simulink model "Test_Nonlinear_system"  (R2022b)
settings: Solver=VariableStepAuto  StartTime=0.0  StopTime=50  RelTol=1e-3
values from neighbouring files (symbols this model uses):
  A = double(A)    [sys_Modelling.m]
  B = double(B)    [sys_Modelling.m]
  C = zeros((N+1)*n, N*p)    [MPC_Matrices.m]    (also in sys_Modelling.m = double(C))
  L = place(sys.A', sys.C',ew_L)'    [Controller_Observer.m]    (also in LQR_Luenberger.m)
undefined symbols (not defined in the file or in its folder): K_neu, u_ap, V_neu
libraries: simulink_extras x2
settings Model: Creator=renzhijian  LastModifiedBy=12056

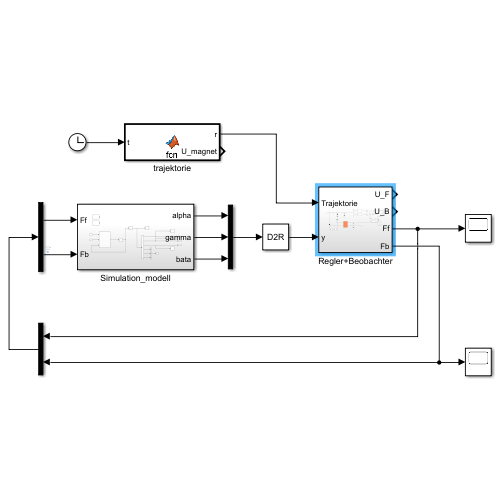
[thumbnail: Simulink's stored preview of the top-level diagram]
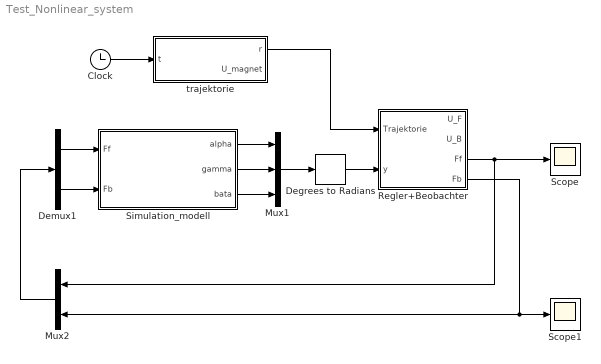
== system Test_Nonlinear_system ==
  Clock : Clock
  Degrees to Radians : simulink_extras/Transformations/Degrees to Radians
  Demux1 : Demux  Outputs=2
  Mux1 : Mux  Inputs=3
  Mux2 : Mux  Inputs=2
  Regler+Beobachter : Subsystem
  Scope : Scope
  Scope1 : Scope
  Simulation_modell : Subsystem
  trajektorie : MATLAB Function  TreatAsAtomicUnit=on
  wires:
  Mux2/1 -> Demux1/1
  Simulation_modell/2(gamma) -> Mux1/2
  Simulation_modell/1(alpha) -> Mux1/1
  Simulation_modell/3(bata) -> Mux1/3
  Regler+Beobachter/3(Ff) -> Scope/1, Mux2/1
  Regler+Beobachter/4(Fb) -> Scope1/1, Mux2/2
  Demux1/1 -> Simulation_modell/1(Ff)
  Demux1/2 -> Simulation_modell/2(Fb)
  Clock/1 -> trajektorie/1(t)
  Mux1/1 -> Degrees to Radians/1
  Degrees to Radians/1 -> Regler+Beobachter/2(y)
  trajektorie/1(r) -> Regler+Beobachter/1(Trajektorie)

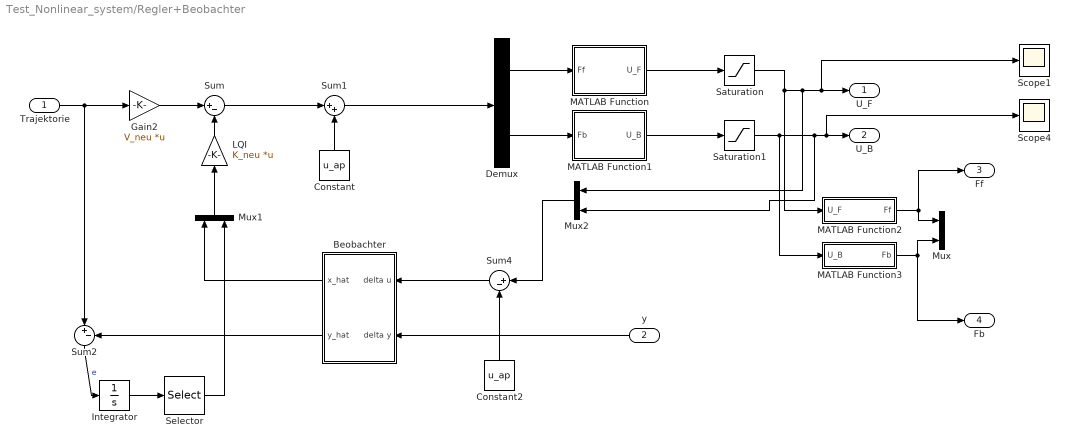
== system Test_Nonlinear_system/Regler+Beobachter ==
  Trajektorie : Inport
  y : Inport  Port=2
  Beobachter : Subsystem
  Constant : Constant  Value=u_ap
  Constant2 : Constant  Value=u_ap
  Demux : Demux  Outputs=2
  Gain2 : Gain  Gain=V_neu  Multiplication=Matrix(K*u) (u vector)
  Integrator : Integrator
  LQI : Gain  Gain=K_neu  Multiplication=Matrix(K*u) (u vector)
  MATLAB Function : MATLAB Function  TreatAsAtomicUnit=on
  MATLAB Function1 : MATLAB Function  TreatAsAtomicUnit=on
  MATLAB Function2 : MATLAB Function  TreatAsAtomicUnit=on
  MATLAB Function3 : MATLAB Function  TreatAsAtomicUnit=on
  Mux : Mux  Inputs=2
  Mux1 : Mux  Inputs=2
  Mux2 : Mux  Inputs=2
  Saturation : Saturate  UpperLimit=4  LowerLimit=0
  Saturation1 : Saturate  UpperLimit=4  LowerLimit=0
  Scope1 : Scope
  Scope4 : Scope
  Selector : Selector  InputPortWidth=3  IndexOptions=Index vector (dialog)  Indices=[1 2]  OutputSizes=1
  Sum : Sum  Inputs=|+-
  Sum1 : Sum  Inputs=|++
  Sum2 : Sum  Inputs=|+-
  Sum4 : Sum  Inputs=|+-
  U_F : Outport
  U_B : Outport  Port=2
  Ff : Outport  Port=3
  Fb : Outport  Port=4
  wires:
  MATLAB Function1/1(U_B) -> Saturation1/1
  y/1 -> Beobachter/2(delta y)
  Saturation1/1 -> Mux2/2, Scope4/1, U_B/1, MATLAB Function3/1(U_B)
  Demux/1 -> MATLAB Function/1(Ff)
  Sum1/1 -> Demux/1
  Saturation/1 -> Mux2/1, Scope1/1, U_F/1, MATLAB Function2/1(U_F)
  MATLAB Function2/1(Ff) -> Ff/1, Mux/1
  MATLAB Function3/1(Fb) -> Fb/1, Mux/2
  Constant2/1 -> Sum4/2
  Constant/1 -> Sum1/2
  MATLAB Function/1(U_F) -> Saturation/1
  Sum4/1 -> Beobachter/1(delta u)
  Demux/2 -> MATLAB Function1/1(Fb)
  Trajektorie/1 -> Gain2/1, Sum2/1
  Sum/1 -> Sum1/1
  Sum2/1 -> Integrator/1  "e"
  Integrator/1 -> Selector/1
  Beobachter/2(y_hat) -> Sum2/2
  Beobachter/1(x_hat) -> Mux1/1
  Mux1/1 -> LQI/1
  LQI/1 -> Sum/2
  Gain2/1 -> Sum/1
  Selector/1 -> Mux1/2
  Mux2/1 -> Sum4/1

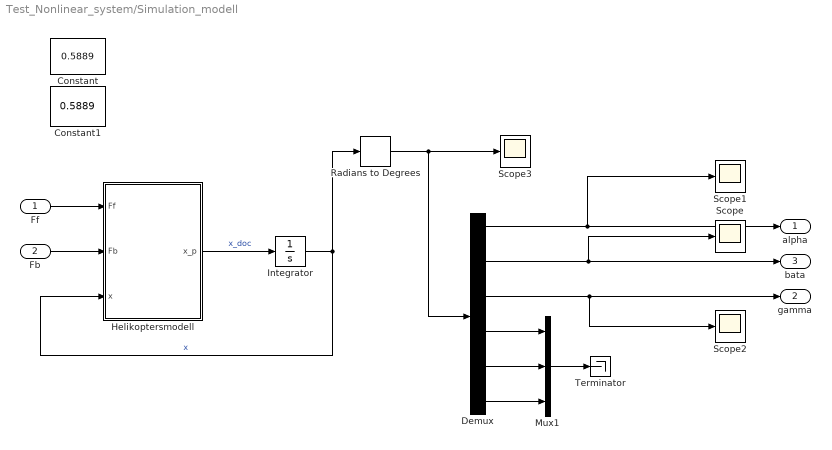
== system Test_Nonlinear_system/Simulation_modell ==
  Ff : Inport
  Fb : Inport  Port=2
  Constant : Constant  Value=0.5889
  Constant1 : Constant  Value=0.5889
  Demux : Demux  Outputs=6
  Helikoptersmodell : MATLAB Function  TreatAsAtomicUnit=on
  Integrator : Integrator  InitialCondition=[0;-27*pi/180;0;0;0;0]
  Mux1 : Mux  Inputs=3
  Radians to Degrees : simulink_extras/Transformations/Radians to Degrees
  Scope{,1..3} (4 alike) : Scope
  Terminator : Terminator
  alpha : Outport  VectorParamsAs1DForOutWhenUnconnected=off
  gamma : Outport  Port=2  VectorParamsAs1DForOutWhenUnconnected=off
  bata : Outport  Port=3  VectorParamsAs1DForOutWhenUnconnected=off
  wires:
  Mux1/1 -> Terminator/1
  Integrator/1 -> Radians to Degrees/1, Helikoptersmodell/3(x)  "x"
  Demux/3 -> Scope2/1, gamma/1
  Radians to Degrees/1 -> Scope3/1, Demux/1
  Demux/4 -> Mux1/1
  Helikoptersmodell/1(x_p) -> Integrator/1  "x_doc"
  Demux/5 -> Mux1/2
  Demux/1 -> Scope1/1, alpha/1
  Demux/2 -> bata/1, Scope/1
  Demux/6 -> Mux1/3
  Ff/1 -> Helikoptersmodell/1(Ff)
  Fb/1 -> Helikoptersmodell/2(Fb)

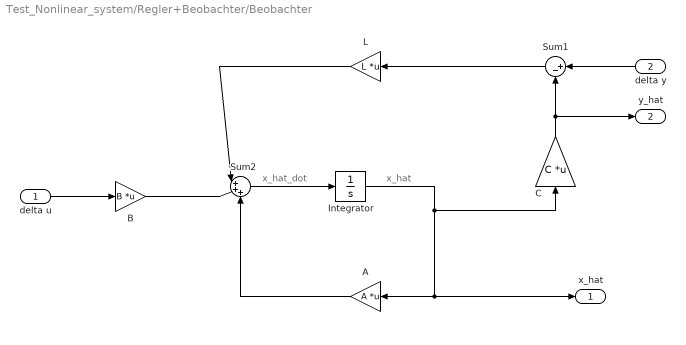
== system Test_Nonlinear_system/Regler+Beobachter/Beobachter ==
  note: x_hat_dot
  note: x_hat
  delta u : Inport
  delta y : Inport  Port=2
  A : Gain  Gain=A  Multiplication=Matrix(K*u) (u vector)
  B : Gain  Gain=B  Multiplication=Matrix(K*u) (u vector)
  C : Gain  Gain=C  Multiplication=Matrix(K*u) (u vector)
  Integrator : Integrator  InitialCondition=[0;-27*pi/180;0;0;0;0]
  L : Gain  Gain=L  Multiplication=Matrix(K*u) (u vector)
  Sum1 : Sum  Inputs=|+-
  Sum2 : Sum  Inputs=|+++
  x_hat : Outport
  y_hat : Outport  Port=2
  wires:
  Integrator/1 -> A/1, x_hat/1, C/1
  L/1 -> Sum2/1
  Sum2/1 -> Integrator/1
  delta u/1 -> B/1
  Sum1/1 -> L/1
  A/1 -> Sum2/3
  B/1 -> Sum2/2
  delta y/1 -> Sum1/1
  C/1 -> Sum1/2, y_hat/1

== matlab function Test_Nonlinear_system/Simulation_modell/Helikoptersmodell ==
  data: Ff input; x_p output; Fb input; x input
function x_p = fcn(Ff, Fb, x)
alpha = x(1);
beta = x(2);
gamma = x(3);
alphadot = x(4);
betadot = x(5);
gammadot = x(6);
%Helikopterseigenschaft
l1 = 0.655; %Distance between travel axis to helicopter body  
l2 = 0.262; %Length of the secondary arm
l3 = 0.1355; %Force arm of the gravity of secondary arm
l4 = 0.2285; %Length from Joint 1 to crossing point
l5 = 0.21; %Length from Joint 1 to midpoint of main arm 
l6 = 0.355/2; %Distance between pitch to each motor 
l7 = 0.534;
h = 0.042+0.019/2; % Distance between axis Y and main arm

%Gewicht
mw = 1.918;%Mass of the counterweight
marm2 = 0.138;%Mass of secondary arm
marm1 = 0.377;%Mass of main arm
mf = 0.661;%Mass of front motor and bodies
mb = 0.661;%Mass of back motor and bodies
mj2 = 0.106;%Mass of the joint2
mmag = 0.07;%Mass of the magnet
g = 9.81;%Erdbeschleunigung
theta = deg2rad(15);%Crossing angle of main and secondary arm
phi = 0.1427;%Deviation of the helicopter relative to joint2
d = 0.102;%Distance between joint3 to the rail

%% MOMENT OF INERTIA
%% beta
J_mw = (1/12)*mw*(0.070^2 + 0.057^2);
J_marm1 = (1/12)*marm1*(0.915^2 + 0.019^2);
J_marm2 = (1/12)*marm2*(0.305^2 + 0.025^2);

Jbeta = J_mw + mw * ((l4+l2*cos(theta))^2+(l2*sin(theta)-h)^2) ...,       % Moment of CounterWeight
    + J_marm1 + marm1 * (((l5)/2)^2+h^2) ...,                               % Moment of main arm
    + J_marm2 + marm2 * (((l3*cos(theta))+l4)^2+(l3*sin(theta)-h)^2) ...,   % Moment of secondary arm
    + (mf+mb)*(l1^2+(0.044+h)^2) ...,                                       % Moment of heli(simplify)
    + mj2*(l1^2+(h+0.019+0.028)^2) ...,                                     % Moment of joint 2
    + mmag*(l7^2+(h+0.062*sin(pi/3))^2);                                    % Moment of Magnet
% 1.1435        1.1708

%% gamma
J_body  =   1/12*0.2*(3*0.114^2 + 0.027^2);           % Body = Cylinder
J_moter =   1/12*0.287*(3*0.0195^2 + 0.069^2);        % Motor = Cylinder
J_bar   =   1/12*0.322*(0.495^2 + 0.006^2);           % Bar = Cubic
J_joint =   1/12*0.026*(0.019^2 + 0.025^2);           % joint = Cubic

Jgamma = 2*(J_body+0.2*((0.027/2+0.069-0.041)^2+(0.355/2)^2))+ ...,           % Moment of bodies
    2*(J_moter+0.287*((0.041-0.069/2)^2+(0.355/2)^2))+ ...,                     % Moment of Motors
    J_bar+0.322*(0.041+0.006/2)^2+ ...,                                         % Moment of bar
    J_joint+0.026*(0.041-0.019/2)^2;                                            % Moment of joints3
% 0.0402        0.0554

%% alpha    simplify
% modification
aRb = [cos(beta) 0 sin(beta); 
    0 1 0; 
    -sin(beta) 0 cos(beta)];
bRc = [cos(gamma) -sin(gamma) 0; 
    sin(gamma) cos(gamma) 0; 
    0 0 1];
arb = [l1*sin(beta); 0; l1*cos(beta)];

cP_f = [-0.065; -l6; 0];
cP_b = [-0.065; l6; 0];

aP_f = aRb*bRc*cP_f + arb;
aP_b = aRb*bRc*cP_b + arb;

D_Pf = aP_f(2)^2 + aP_f(3)^2;
D_Pb = aP_b(2)^2 + aP_b(3)^2;


J_mw_alpha = (1/12)*mw*((0.070^2 + 0.057^2)*(sin((pi/2)+beta-theta))^2+(0.057^2 + 0.057^2)*(cos((pi/2)+beta-theta))^2);
J_marm1_alpha = (1/12)*marm1*((0.915^2+0.019^2)*(cos(beta))^2+(0.019^2+0.019^2)*(sin(beta))^2);
J_marm2_alpha = (1/12)*marm2*((0.305^2+0.025^2)*(cos(beta-theta))^2 +(0.025^2+0.025^2)*(sin(beta-theta))^2);
J_j1_alpha = 1/12*0.029*((0.019^2 + 0.025^2)*(cos(beta))^2 + (0.019^2 + 0.019^2)*(sin(beta))^2);
J_bar_alpha =  1/12*0.322*((0.495^2 + 0.006^2)*((cos(beta))^2+(cos(gamma))^2) + (0.006^2 + 0.006^2)*(sin(beta))^2);
J_joint_alpha =   1/12*0.026*((0.019^2 + 0.025^2)*((cos(beta))^2+(cos(gamma))^2) + (0.019^2 + 0.019^2)*(sin(beta))^2);
J_body_alpha = 1/12*0.2*(3*0.114^2 + 0.027^2)*((sin(beta))^2+(cos(gamma))^2) + 1/2*0.2*0.114^2*(cos(beta))^2; 
J_moter_alpha =   1/12*0.287*(3*0.0195^2 + 0.069^2)*((sin(beta))^2+(cos(gamma))^2) + 1/2*0.287*0.0195^2*(cos(beta))^2;

Jalpha = J_mw_alpha + mw*((l4*cos(beta)+l2*cos(theta-beta))^2) ...,                  % Moment of CounterWeight
    + J_marm1_alpha + marm1*(l5*cos(beta))^2 ...,                                    % Moment of main arm
    + J_marm2_alpha + marm2*((l3*cos(theta-beta)+l4*cos(beta))^2)...,               % Moment of secondary arm
    + mj2*(l1*cos(beta))^2 ...,                                                % Moment of joint2
    + mmag*(l7*cos(beta))^2 ...,                                               % Moment of magnet
    + J_j1_alpha + 0.029*((0.042-0.019/2)*sin(beta))^2 ...,                          % Moment of joint1
    + J_bar_alpha + 0.322*(l1*cos(beta)+(0.042+0.019+0.028+0.041+0.006/2)*sin(beta))^2 ...,  % Moment of bar
    + J_joint_alpha + 0.026*(l1*cos(beta)+(0.042+0.019+0.028+0.041-0.019/2)*sin(beta))^2 ...,% Moment of joint3
    + 2*J_body_alpha + 2*J_moter_alpha + (0.2+0.287)*(D_Pf+D_Pb);                           % Moment of Motors and Bodies
% 1.1794

%% MOMENT
%% alpha
Malpha = -(Ff+Fb)*sin(gamma)*l1*cos(beta);

%% beta
M_all = (mw*g*(l2*cos(theta)+l4) + marm2*g*(l3*cos(theta)+l4) - (mf+mb+mj2)*g*l1 - marm1*g*l5 -mmag*g*l7)*cos(0);
mass_position = M_all / ((mw+marm2+marm1+mmag+mj2+mf+mb)*g);
Mbeta = (Ff+Fb)*l1*cos(gamma) + (mw+marm2+marm1+mmag+mj2+mf+mb)*g*(mass_position*cos(beta)-h*sin(beta));

%% gamma
Mgamma = (Ff-Fb)*l6 + mb*g*cos(phi+gamma)*l6/cos(phi) - mf*g*cos(phi-gamma)*l6/cos(phi);




%% SOLVE
alphadot_2 = Malpha/Jalpha;
betadot_2 = Mbeta/Jbeta;        % 1.1435
gammadot_2 = Mgamma/Jgamma;     % 0.0402


x_p = [alphadot;
    betadot;
    gammadot;
    alphadot_2;
    betadot_2;
    gammadot_2
    ];
x_p(1:3) = x(4:6);
x_p(4) = alphadot_2;
x_p(5) = betadot_2;
x_p(6) = gammadot_2;

== matlab function Test_Nonlinear_system/Regler+Beobachter/MATLAB Function ==
  data: Ff input; U_F output
function U_F = fcn(Ff)
 U_F= (10000/733*abs(Ff))^(1/2);
end

== matlab function Test_Nonlinear_system/Regler+Beobachter/MATLAB Function1 ==
  data: Fb input; U_B output
function U_B = fcn(Fb)
 U_B= sqrt(1000/66*abs(Fb));
end

== matlab function Test_Nonlinear_system/Regler+Beobachter/MATLAB Function2 ==
  data: U_F input; Ff output
function Ff = fcn(U_F)
Ff = 0.0733*U_F^2;
end

== matlab function Test_Nonlinear_system/Regler+Beobachter/MATLAB Function3 ==
  data: U_B input; Fb output
function Fb = fcn(U_B)
 Fb = 0.066*U_B^2;
end

== matlab function Test_Nonlinear_system/trajektorie ==
  data: t input; r output; U_magnet output
function [r, U_magnet] = fcn(t)
beta = -27;
if t <= 10
    a0 = five_times_plan(0, -27, 0, 0, 10, 0, 0, 0);
    alpha = 0;
    beta = a0(1)+a0(2)*t+a0(3)*t^2+a0(4)*t^3+a0(5)*t^4+a0(6)*t^5;
    U_magnet = 0;
elseif t > 10 && t <= 18
    a0 = five_times_plan(10, 0, 0, 0, 18, 90, 0, 0);
    alpha = a0(1)+a0(2)*t+a0(3)*t^2+a0(4)*t^3+a0(5)*t^4+a0(6)*t^5;
    beta = 0;
    U_magnet = 0;
elseif t > 18 &&t <= 26
    a0 = five_times_plan(18, 0, 0, 0, 26, -22, 0, 0);
    alpha = 90;
    beta = a0(1)+a0(2)*t+a0(3)*t^2+a0(4)*t^3+a0(5)*t^4+a0(6)*t^5;
    U_magnet = 1;
elseif t > 26 && t <= 30
    alpha = 90;
    beta = -22;
    U_magnet = 0;
elseif t > 30 && t <= 38
    a0 = five_times_plan(30, -22, 0, 0, 38, 0, 0, 0);
    alpha = 90;
    beta = a0(1)+a0(2)*t+a0(3)*t^2+a0(4)*t^3+a0(5)*t^4+a0(6)*t^5;
    U_magnet = 0;
elseif t > 38 && t <= 62
    a0 = five_times_plan(38, 90, 0, 0,62, 450, 0, 0);
    alpha = a0(1)+a0(2)*t+a0(3)*t^2+a0(4)*t^3+a0(5)*t^4+a0(6)*t^5;
    beta = 0;
    U_magnet = 0;
elseif t > 62 && t <= 70
    a0 = five_times_plan(62, 0, 0, 0, 70, -22, 0, 0); 
    alpha = 450;
    beta = a0(1)+a0(2)*t+a0(3)*t^2+a0(4)*t^3+a0(5)*t^4+a0(6)*t^5;
    U_magnet = 1;
elseif t > 70 && t <= 74
    alpha = 450;
    beta = -22;
    U_magnet = 0;
elseif t > 74 && t <= 82
    a0 = five_times_plan(74, -22, 0, 0, 82, 0, 0, 0);
    alpha = 450;
    beta = a0(1)+a0(2)*t+a0(3)*t^2+a0(4)*t^3+a0(5)*t^4+a0(6)*t^5;
    U_magnet = 0;
elseif t > 82 && t <= 110
    a0 = five_times_plan(82, 450, 0, 0, 110, 0, 0, 0);
    alpha = a0(1)+a0(2)*t+a0(3)*t^2+a0(4)*t^3+a0(5)*t^4+a0(6)*t^5;
    beta = 0;
    U_magnet = 0;
elseif t > 110 && t < 118
    a0 = five_times_plan(110, 0, 0, 0, 118, -27, 0, 0);
    alpha = 0;
    beta = a0(1)+a0(2)*t+a0(3)*t^2+a0(4)*t^3+a0(5)*t^4+a0(6)*t^5;
    U_magnet = 1;
else 
    alpha = 0; beta = -27;
    U_magnet = 0;
end
r = [alpha; beta;0];
function a = five_times_plan(ts, xs, vs, as, te, xe, ve, ae)
    para = [xs;vs;as;xe;ve;ae];
    Tran = [1,   ts,  ts^2,  ts^3,    ts^4,     ts^5;
            0,   1,   2*ts,  3*ts^2,  4*ts^3,   5*ts^4;
            0,   0,   2,     6*ts,    12*ts^2,  20*ts^3;
            1,   te,  te^2,  te^3,    te^4,     te^5;
            0,   1,   2*te,  3*te^2,  4*te^3,   5*te^4;
            0,   0,   2,     6*te,    12*te^2,  20*te^3];
    a = inv(Tran)*para;
end
end
